simulink library "alfa_floor"  (R2018b)
settings: Solver=ode45  StartTime=0.0  StopTime=10.0  RelTol=1e-3  EnableMultiTasking=on
settings Model: Creator=lena.frank  LastModifiedBy=drhf
settings DataIOCC: LimitDataPoints=on  SaveFormat=Array  SignalLoggingSaveFormat=ModelDataLogs
settings OptimizationCC: ExpressionDepthLimit=2147483647  LifeSpan=inf
settings DebuggingCC: UnderspecifiedInitializationDetection=Classic  MergeDetectMultiDrivingBlocksExec=none  SolverPrmCheckMsg=warning  FcnCallInpInsideContextMsg=warning  StateNameClashWarn=warning  SFUnexpectedBacktrackingDiag=warning  SFNoUnconditionalDefaultTransitionDiag=warning  SFExecutionAtInitializationDiag=none
settings HardwareCC: ProdBitPerPointer=32  ProdBitPerSizeT=32  ProdBitPerPtrDiffT=32  ProdLargestAtomicFloat=None  ProdIntDivRoundTo=Undefined  ProdEndianess=Unspecified  ProdWordSize=32  ProdHWDeviceType=32-bit Generic
settings ModelReferenceCC: PropagateSignalLabelsOutOfModel=off
settings SFSimCC: SimUseLocalCustomCode=off
settings RTWCC: RTWUseLocalCustomCode=off
settings CodeAppCC: StateflowObjectComments=on
settings GRTTargetCC: TargetLangStandard=C89/C90 (ANSI)  GeneratePreprocessorConditionals=Disable all  CombineOutputUpdateFcns=off  GRTInterface=on
settings ConfigComp: CovMetricSettings=dw  CovHtmlReporting=on  CovSaveCumulativeToWorkspaceVar=on  CovSaveSingleToWorkspaceVar=on  CovExternalEMLEnable=off

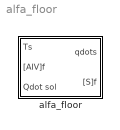
== system alfa_floor ==
  alfa_floor : Subsystem  mask(ALFA){active=0, emission_f=0.65, wallsurface=1}
      mask prompts: active "active layer (0 / 1)"; emission_f "Longwave emissivity of surface (0..1)"; wallsurface "Floor surface in m²"
      mask help:
      | Convective and radiative heat transfer at the SURFACE OF A HORIZONTAL FLOOR.
      |
      | [AIV] : conditions of zone node,
      | Ts : temperature of wall surface, °C,
      | qdots : specific heat flow into wall construction, W/m^2,
      | [S] : heat and air flow to zone node.
      mask Help: web(fullfile(path_carnot('help'),'alfa_floor.html'),'-helpbrowser')

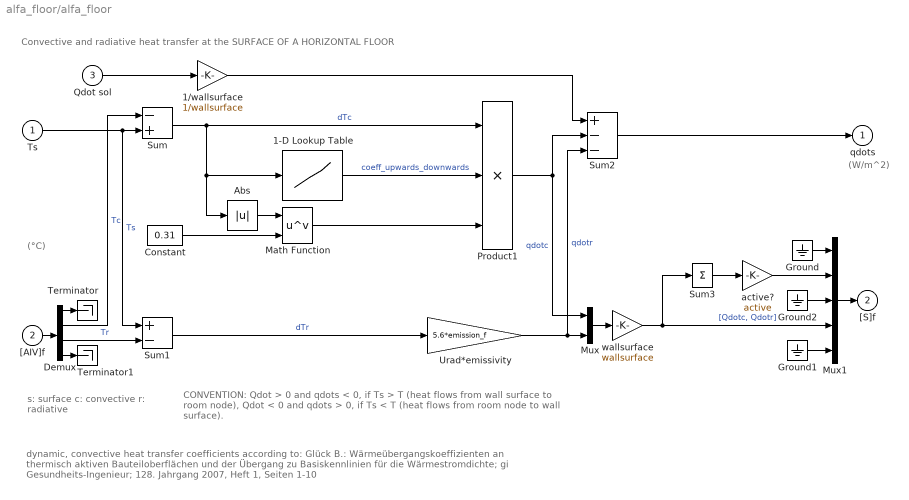
== system alfa_floor/alfa_floor ==
  note: CONVENTION:
      | Qdot > 0 and qdots < 0, if Ts > T (heat flows from wall surface to room node),
      | Qdot < 0 and qdots > 0, if Ts < T (heat flows from room node to wall surface).
  note: s: surface
      | c: convective
      | r: radiative
  note: Convective and radiative heat transfer at the SURFACE OF A HORIZONTAL FLOOR
  note: (W/m^2)
  note: (°C)
  note: dynamic, convective heat transfer coefficients according to: Glück B.: Wärmeübergangskoeffizienten an thermisch aktiven Bauteiloberflächen
      | und der Übergang zu Basiskennlinien für die Wärmestromdichte; gi Gesundheits-Ingenieur; 128. Jahrgang 2007, Heft 1, Seiten 1-10
  Ts : Inport
  "[AIV]f" : Inport  Port=2
  Qdot sol : Inport  Port=3
  1-D Lookup Table : Lookup_n-D  NumberOfTableDimensions=1  BreakpointsForDimension1=[-10 -0.01 0.01 10]  BeginIndexSearchUsingPreviousIndexResult=on  Table=[0.54 0.54 2 2]  InternalRulePriority=Speed  RndMeth=Simplest  InputSameDT=on
  1/wallsurface : Gain  Gain=1/wallsurface  SaturateOnIntegerOverflow=on  OutDataTypeStr=Inherit: Same as input  ParamDataTypeStr=Inherit: Same as input
  Abs : Abs
  Constant : Constant  Value=0.31
  Demux : Demux  Outputs=[1 1 1 6]
  Ground : Ground
  Ground1 : Ground
  Ground2 : Ground
  Math Function : Math  Operator=pow  SaturateOnIntegerOverflow=on
  Mux : Mux  Inputs=[1 1]
  Mux1 : Mux  Inputs=[4 1 1 2 5]
  Product1 : Product  Inputs=3  SaturateOnIntegerOverflow=on  RndMeth=Zero  InputSameDT=on  OutDataTypeStr=Inherit: Same as first input
  Sum : Sum  Inputs=-+  SaturateOnIntegerOverflow=on  InputSameDT=on  OutDataTypeStr=Inherit: Same as first input
  Sum1 : Sum  Inputs=+-  SaturateOnIntegerOverflow=on  InputSameDT=on  OutDataTypeStr=Inherit: Same as first input
  Sum2 : Sum  Inputs=+--  SaturateOnIntegerOverflow=on  InputSameDT=on  OutDataTypeStr=Inherit: Same as first input
  Sum3 : Sum  Inputs=1  SaturateOnIntegerOverflow=on  InputSameDT=on  OutDataTypeStr=Inherit: Same as first input
  Terminator : Terminator
  Terminator1 : Terminator
  Urad*emissivity : Gain  Gain=5.6*emission_f  SaturateOnIntegerOverflow=on  OutDataTypeStr=Inherit: Same as input  ParamDataTypeStr=Inherit: Same as input
  active? : Gain  Gain=active  SaturateOnIntegerOverflow=on  OutDataTypeStr=Inherit: Same as input  ParamDataTypeStr=Inherit: Same as input
  wallsurface : Gain  Gain=wallsurface  SaturateOnIntegerOverflow=on  OutDataTypeStr=Inherit: Same as input  ParamDataTypeStr=Inherit: Same as input
  qdots : Outport
  "[S]f" : Outport  Port=2
  wires:
  active?/1 -> Mux1/2
  Ground2/1 -> Mux1/3
  Mux1/1 -> "[S]f"/1
  Ground1/1 -> Mux1/5
  Ground/1 -> Mux1/1
  Sum3/1 -> active?/1
  Qdot sol/1 -> 1/wallsurface/1
  wallsurface/1 -> Sum3/1, Mux1/4  "[Qdotc, Qdotr]"
  Demux/2 -> Sum/1  "Tc"
  Sum2/1 -> qdots/1
  Ts/1 -> Sum/2, Sum1/1  "Ts"
  1/wallsurface/1 -> Sum2/1
  Demux/4 -> Terminator1/1
  "[AIV]f"/1 -> Demux/1
  Demux/1 -> Terminator/1
  Sum1/1 -> Urad*emissivity/1  "dTr"
  Urad*emissivity/1 -> Mux/2, Sum2/3  "qdotr"
  Mux/1 -> wallsurface/1
  Product1/1 -> Sum2/2, Mux/1  "qdotc"
  Demux/3 -> Sum1/2  "Tr"
  Math Function/1 -> Product1/3
  1-D Lookup Table/1 -> Product1/2  "coeff_upwards_downwards"
  Abs/1 -> Math Function/1
  Constant/1 -> Math Function/2
  Sum/1 -> Abs/1, 1-D Lookup Table/1, Product1/1  "dTc"
